simulink model "Tiempos_servicio"  (R2023a)
settings: Solver=VariableStepAuto  StartTime=0.0  StopTime=20  RelTol=1e-3
undefined symbols (not defined in the file): m, n
libraries: simulink x1
settings Model: Creator=santi  LastModifiedBy=santi

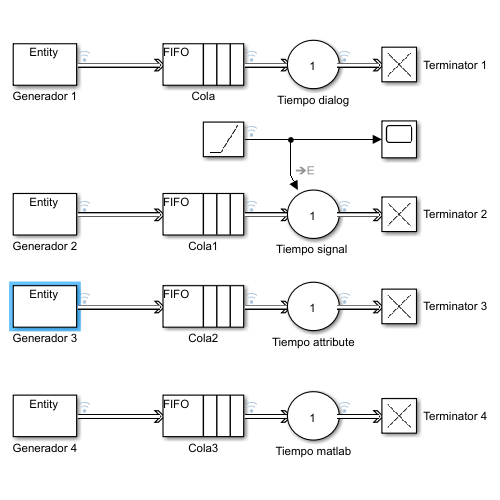
[thumbnail: Simulink's stored preview of the top-level diagram]
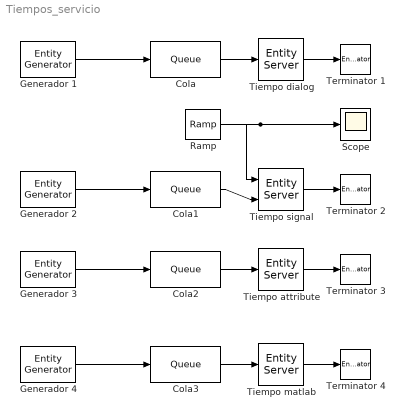
== system Tiempos_servicio ==
  Cola{,1..3} (4 alike) : Queue  InputPortMessageModes=m  OutputPortMessageModes=m
  Generador 1 : EntityGenerator  OutputPortMessageModes=m  EntityType=Structured  EntityTypeName=Entity
  Generador 2 : EntityGenerator  OutputPortMessageModes=m  EntityType=Structured  EntityTypeName=Entity
  Generador 3 : EntityGenerator  OutputPortMessageModes=m  AttributeInitialValue=4  EntityType=Structured  EntityTypeName=Entity
  Generador 4 : EntityGenerator  OutputPortMessageModes=m  EntityType=Structured  EntityTypeName=Entity
  Ramp : simulink/Sources/Ramp  slope=1  start=0  InitialOutput=0
  Scope : Scope
  Terminator {1..4} (4 alike) : EntityTerminator  InputPortMessageModes=m
  Tiempo attribute : EntityServer  InputPortMessageModes=m  OutputPortMessageModes=m  Capacity=1  ServiceTimeSource=Attribute  ServiceTimeValue=2  ServiceTimeAttributeName=Attribute1
  Tiempo dialog : EntityServer  InputPortMessageModes=m  OutputPortMessageModes=m  Capacity=1  ServiceTimeValue=2
  Tiempo matlab : EntityServer  InputPortMessageModes=m  OutputPortMessageModes=m  Capacity=1  ServiceTimeValue=2
  "Tiempo signal " : EntityServer  InputPortMessageModes=n,m  OutputPortMessageModes=m  Capacity=1  ServiceTimeSource=Signal port  ServiceTimeValue=2
      settings: InputPortMap=u0,u2
  wires:
  Generador 1/1 -> Cola/1
  Cola/1 -> Tiempo dialog/1
  Tiempo dialog/1 -> Terminator 1/1
  "Tiempo signal "/1 -> Terminator 2/1
  Cola1/1 -> "Tiempo signal "/2
  Generador 2/1 -> Cola1/1
  Generador 3/1 -> Cola2/1
  Cola2/1 -> Tiempo attribute/1
  Tiempo attribute/1 -> Terminator 3/1
  Tiempo matlab/1 -> Terminator 4/1
  Cola3/1 -> Tiempo matlab/1
  Generador 4/1 -> Cola3/1
  Ramp/1 -> "Tiempo signal "/1, Scope/1
